simulink model "fault"  (R2017b)
settings: Solver=VariableStepAuto  StartTime=0.0  StopTime=1  MaxStep=1e-4  RelTol=1e-3
undefined symbols (not defined in the file): D1, Delta
libraries: powerlib x10
settings Model: Creator=cheeku.triven  LastModifiedBy=cheeku.triven

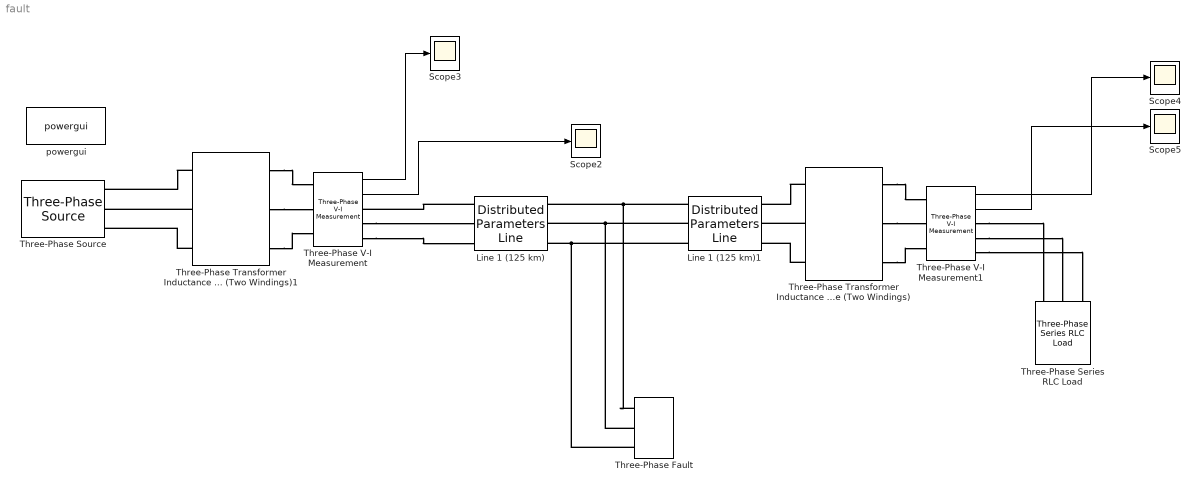
== system fault ==
  Line 1 (125 km) : powerlib/Elements/Distributed Parameters Line  Phases=3  Frequency=50  Resistance=[0.01273 0.3868]  Inductance=[0.9337e-3 4.1264e-3]  Capacitance=[12.74e-9 7.751e-9]  Length=125  x1=[1.59467191624238e-07 16183.8339204588 16183.8339205328;314.159265358979 314.159265358979 314.159265358979;-0.616279923585432 -2.32608069025364 2.38630829012418]  x2=[1.61244074655788e-07 16577.1628154969 16577.1628155711;314.159265358979 314.159265358979 314.159265358979;-0.605279074187556 -2.32908665287446 2.38330232750356]  x3=[2.22725144977065e-10 60.4650474678237 60.4650474681747;314.159265358979 314.159265358979 314.159265358979;-0.753244686847752 -2.57349483887261 2.13889414150632]  x4=[1.98400696917289e-10 62.179657633283 62.1796576334704;314.159265358979 314.159265358979 314.159265358979;-0.68994921536332 -2.22230910272841 2.49007987764901]  x5=0.000706926958744678  V1=[1.595e-07 1.618e+04 1.618e+04;314.2 314.2 314.2;-0.6163 -2.326 2.386]  V2=[1.612e-07 1.658e+04 1.658e+04;314.2 314.2 314.2;-0.6053 -2.329 2.383]  I1=[2.227e-10 60.47 60.47;314.2 314.2 314.2;-0.7532 -2.573 2.139]  I2=[1.984e-10 62.18 62.18;314.2 314.2 314.2;-0.6899 -2.222 2.49]  nHarmo=1  Measurements=Phase-to-ground voltages
      settings: AttributesFormatString=\n  SourceProductName=Simscape Power Systems
  Line 1 (125 km)1 : powerlib/Elements/Distributed Parameters Line  Phases=3  Frequency=50  Resistance=[0.01273 0.3864]  Inductance="[0.9337e-3  4.1264e-3]"  Capacitance=[12.74e-9 7.751e-9]  Length=125  x1=[1.61243904634339e-07 16577.1628154969 16577.1628155711;314.159265358979 314.159265358979 314.159265358979;-0.605276458477394 -2.32908665287446 2.38330232750356]  x2=[1.5517083249881e-07 16666.99821671 16666.998216783;314.159265358979 314.159265358979 314.159265358979;-0.578599986777585 -2.33117972382874 2.38120925654947]  x3=[2.23812802839206e-10 60.4841629286646 60.4841629290158;314.159265358979 314.159265358979 314.159265358979;-0.529788916282644 -2.43886931217874 2.2735196682002]  x4=[1.98732606876864e-10 62.1559384797901 62.1559384799783;314.159265358979 314.159265358979 314.159265358979;-0.902391780234354 -2.35814348311034 2.35424549726709]  x5=0.000706926958744678  V1=[1.612e-07 1.658e+04 1.658e+04;314.2 314.2 314.2;-0.6053 -2.329 2.383]  V2=[1.552e-07 1.667e+04 1.667e+04;314.2 314.2 314.2;-0.5786 -2.331 2.381]  I1=[2.238e-10 60.48 60.48;314.2 314.2 314.2;-0.5298 -2.439 2.274]  I2=[1.987e-10 62.16 62.16;314.2 314.2 314.2;-0.9024 -2.358 2.354]  nHarmo=1  Measurements=Phase-to-ground voltages
      settings: AttributesFormatString=\n  SourceProductName=Simscape Power Systems
  Scope{2..5} (4 alike) : Scope
  Three-Phase Series RLC Load : powerlib/Elements/Three-Phase Series RLC Load  LConnTagsString=A|B|C  Configuration=Y (grounded)  NominalVoltage=138e2  Vabc=[1e3 1e3 1e3]  Vabcp=[1e3 1e3 1e3]  NominalFrequency=50  UnbalancedPower=off  ActivePower=10e6  InductivePower=1000  CapacitivePower=100  Pabc=[10e3 9e3 11e3]  QLabc=[100 90 110]  QCabc=[100 90 110]  Pabcp=[10e3 9e3 11e3]  QLabcp=[100 90 110]  QCabcp=[100 90 110]  Measurements=None  LoadType=constant Z
  Three-Phase V-I Measurement : powerlib/Measurements/Three-Phase V-I Measurement  VoltageMeasurement=phase-to-ground  SetLabelV=off  LabelV=Vabc  Vpu=on  VpuLL=off  CurrentMeasurement=yes  SetLabelI=off  LabelI=Iabc  Ipu=on  Pbase=100e6  Vbase=115e3  OutputType=Complex  PhasorSimulation=off  PSBequivalent=0
  Three-Phase V-I Measurement1 : powerlib/Measurements/Three-Phase V-I Measurement  VoltageMeasurement=phase-to-ground  SetLabelV=off  LabelV=Vabc  Vpu=on  VpuLL=off  CurrentMeasurement=yes  SetLabelI=off  LabelI=Iabc  Ipu=on  Pbase=100e6  Vbase=138e2  OutputType=Complex  PhasorSimulation=off  PSBequivalent=0
  Three-Phase Fault : powerlib/Elements/Three-Phase Fault  InitialStates=0  FaultA=on  FaultB=on  FaultC=on  GroundFault=on  SwitchTimes="[1/50  5/50]"  External=off  SwitchStatus=NaN  FaultResistance=0.001  GroundResistance=0.01  SnubberResistance=1e6  SnubberCapacitance=inf  Measurements=None
  Three-Phase Source : powerlib/Electrical Sources/Three-Phase Source  InternalConnection=Yg  VoltagePhases=off  Voltage=138e2  PhaseAngle=0  Voltage_phases=[25e3 25e3 25e3]/sqrt(3)  PhaseAngles_phases=[0 -120 +120]  Frequency=50  NonIdealSource=on  SpecifyImpedance=off  Resistance=0.8929  Inductance=16.58e-3  ShortCircuitLevel=100e6  BaseVoltage=15e3  XRratio=7  BusType=swing  Pref=10e3  Qref=0  Prefabc=[10e3, 10e3, 10e3]  Qrefabc=[0, 0, 0]  Qmin=-inf  Qmax=inf
  Three-Phase Transformer Inductance Matrix Type (Two Windings) : powerlib/Elements/Three-Phase Transformer Inductance Matrix Type (Two Windings)  CoreType=Three-limb or five-limb core  Winding1Connection=Delta (D1)  Winding2Connection=Yg  AutoTransformer=off  Measurements=None  NominalPower=[15e6, 50]  VLLnom=[115e3,138e2]  WindingResistances=[0.01, 0.01]  NoLoadIexcPos=2  NoLoadPlossPos=1000  ShortCircuitReactancePos=0.06  ShortCircuitReactancePosAuto=0.06  NoLoadIexcZero=100  NoLoadPlossZero=1500  ShortCircuitReactanceZero=0.03  ShortCircuitReactanceZeroAuto=0.03
      settings: SourceProductName=Simscape Power Systems  SourceProductBaseCode=PS
  Three-Phase Transformer Inductance Matrix Type (Two Windings)1 : powerlib/Elements/Three-Phase Transformer Inductance Matrix Type (Two Windings)  CoreType=Three single-phase cores  Winding1Connection=Yg  Winding2Connection=Delta (D1)  AutoTransformer=off  Measurements=None  NominalPower=[15e6, 50]  VLLnom=[138e2, 115e3]  WindingResistances=[0.01, 0.01]  NoLoadIexcPos=0.1  NoLoadPlossPos=1500  ShortCircuitReactancePos=0.06  ShortCircuitReactancePosAuto=0.06  NoLoadIexcZero=100  NoLoadPlossZero=1500  ShortCircuitReactanceZero=0.03  ShortCircuitReactanceZeroAuto=0.03
      settings: SourceProductName=Simscape Power Systems  SourceProductBaseCode=PS
  powergui : powerlib/powergui  Priority=1  SimulationMode=Continuous  SampleTime=50e-6  frequency=60  Iterations=50  frequencyindice=50  Pbase=100e6  ErrMax=1e-4  UnitsV=kV  UnitsW=MW  buscounter=0  FunctionMessages=off  echomessages=off  EnableUseOfTLC=off  CurrentSourceSwitches=off  DisableSnubberDevices=off  DisableRonSwitches=off  DisableVfSwitches=off  DisplayEquations=off  SolverType=Tustin/Backward Euler (TBE)  Interpol=off  ExternalGateDelay=off  methode=off  Ts=100  x0status=blocks  SPID=on  SwTol=0  HookPort=off  RestoreLinks=warning  ResistiveCurrentMeasurement=off  Frange=[0:2:500]  Ylog=off  Xlog=on  ShowGrid=off  save=off  variable=ZData  structure=0  ZoomFFT=off  StartTime=0.0  cycles=1  DisplayStyle=1  fundamental=60  FreqAxis=off  MaxFrequency=1000  frequencyindicesteady=1  RmsSteady=1  display=off
  wires:
  Three-Phase V-I Measurement1/2 -> Scope5/1
  Three-Phase V-I Measurement1/1 -> Scope4/1
  Three-Phase V-I Measurement/1 -> Scope3/1
  Three-Phase V-I Measurement/2 -> Scope2/1
  connections:
  Three-Phase Transformer Inductance Matrix Type (Two Windings)1/LConn1 -- Three-Phase Source/RConn1
  Three-Phase Transformer Inductance Matrix Type (Two Windings)1/LConn2 -- Three-Phase Source/RConn2
  Three-Phase Transformer Inductance Matrix Type (Two Windings)1/LConn3 -- Three-Phase Source/RConn3
  Three-Phase Transformer Inductance Matrix Type (Two Windings)1/RConn1 -- Three-Phase V-I Measurement/LConn1
  Three-Phase Transformer Inductance Matrix Type (Two Windings)1/RConn2 -- Three-Phase V-I Measurement/LConn2
  Three-Phase Transformer Inductance Matrix Type (Two Windings)1/RConn3 -- Three-Phase V-I Measurement/LConn3
  Line 1 (125 km)/LConn1 -- Three-Phase V-I Measurement/RConn1
  Three-Phase V-I Measurement/RConn2 -- Line 1 (125 km)/LConn2
  Three-Phase V-I Measurement/RConn3 -- Line 1 (125 km)/LConn3
  Line 1 (125 km)1/LConn1 -- Three-Phase Fault/LConn1 -- Line 1 (125 km)/RConn1
  Line 1 (125 km)1/LConn2 -- Three-Phase Fault/LConn2 -- Line 1 (125 km)/RConn2
  Line 1 (125 km)1/LConn3 -- Three-Phase Fault/LConn3 -- Line 1 (125 km)/RConn3
  Three-Phase Transformer Inductance Matrix Type (Two Windings)/LConn1 -- Line 1 (125 km)1/RConn1
  Three-Phase Transformer Inductance Matrix Type (Two Windings)/LConn2 -- Line 1 (125 km)1/RConn2
  Three-Phase Transformer Inductance Matrix Type (Two Windings)/LConn3 -- Line 1 (125 km)1/RConn3
  Three-Phase Transformer Inductance Matrix Type (Two Windings)/RConn1 -- Three-Phase V-I Measurement1/LConn1
  Three-Phase Transformer Inductance Matrix Type (Two Windings)/RConn2 -- Three-Phase V-I Measurement1/LConn2
  Three-Phase Transformer Inductance Matrix Type (Two Windings)/RConn3 -- Three-Phase V-I Measurement1/LConn3
  Three-Phase V-I Measurement1/RConn1 -- Three-Phase Series RLC Load/LConn1
  Three-Phase V-I Measurement1/RConn2 -- Three-Phase Series RLC Load/LConn2
  Three-Phase V-I Measurement1/RConn3 -- Three-Phase Series RLC Load/LConn3
